simulink library "dlbsBlockSquare"  (R2025b)
settings: Solver=VariableStepAuto  StartTime=0.0  StopTime=10.0  RelTol=1e-3
libraries: dlbsBlockExtractGradientGF x1, dlbsBlockInsertGradientGF x1
settings Model: Creator=lt6037  LastModifiedBy=lt6037

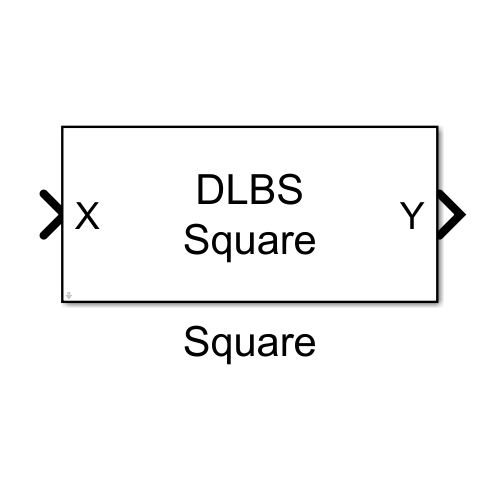
[thumbnail: Simulink's stored preview of the top-level diagram]
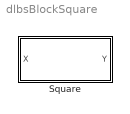
== system dlbsBlockSquare ==
  Square : Subsystem
      mask help: Squares the input tensor. The operation is applied element-wise across all tensor elements.
      mask Help: web("dlbsHelpBlockSquare.html")
      mask Display: fprintf("DLBS\nSquare");

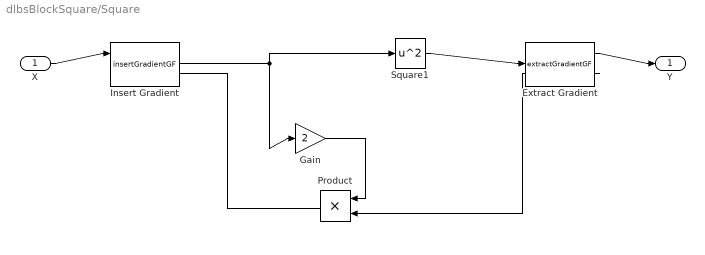
== system dlbsBlockSquare/Square ==
  X : Inport
  Extract Gradient : dlbsBlockExtractGradientGF/extractGradientGF
  Gain : Gain  Gain=2
  Insert Gradient : dlbsBlockInsertGradientGF/insertGradientGF
  Product : Product
  Square1 : Math  Operator=square
  Y : Outport
  wires:
  Gain/1 -> Product/1
  Insert Gradient/1 -> Gain/1, Square1/1
  Square1/1 -> Extract Gradient/1
  Extract Gradient/2 -> Product/2
  Product/1 -> Insert Gradient/2
  Extract Gradient/1 -> Y/1
  X/1 -> Insert Gradient/1
